simulink model "b10_wp_snake"  (R2021b)
settings: Solver=VariableStepAuto  StartTime=0.0  StopTime=Inf  FixedStep=sampleTime  RelTol=1e-3  EnableMultiTasking=on
InitFcn:
  | sampleTime = 0.05;
  | nMedianSize=3;
  | % Robot parameters
  | % Robot parameters
  | wheelRadius = 0.0303;
  | robotRadius = 0.07;   %小车在仿真中显示的圆形的半径大小
  | Trackwidth = 0.0847;  %定义向量场直方图算法中小车的宽度
  | 
  | % Lidar parameters
  | sensorOffset = [0,0];
  | scanAngles = linspace(-pi/3,pi/3,20)';%y = linspace(x1,x2,n) 生成 n 个点。这些点的间距为 (x2-x1)/(n-1)。
  | maxRange = 0.2;
  | 
  | %%%%%%
  | ks=1;
  | 
  | init_pose_1=[0    0  0]';
  | init_pose_2=[0    0.2  -pi/2]';
  | init_pose_3=[0    0.4  -pi/2]';
  | init_pose_4=[0    0.6  -pi/2]';
  | init_pose_5=[0    0.8  -pi/2]';
  | init_pose_6=[0    1  -pi/2]';
  | init_pose_7=[0    1.2  -pi/2]';
  | init_pose_8=[0    1.4  -pi/2]';
  | init_pose_9=[0    1.6  -pi/2]';
  | init_pose_10=[0   1.8  -pi/2]';
  | 
  | % paremeters of pure persuit
  | desired_v=0.2;
  | desired_w=2*pi;
  | desired_lookahead=0.2;
  | kv=0;
  | kw=1;%加速转弯
  | GoalRadius=0.15;%到达目标判定阈值
  | 
  | % paremeters of recovery
  | %recovery_w=0.5
  | recovery_w=2;
  | % Vector Field Histogram
  | numSector=180;%Number of angular sector
  | vehicleRadius=robotRadius;
  | rangeDis=[ 0, 0 ];%Range distance limits (m):
  | thresholds=[ 3, 8 ];%Histogram thresholds
  | %binary histogram 大于8是障碍物，小于3是空白区
  | %Thresholds for computing binary histogram, specified as a two-element vector of scalars. The algorithm uses these thresholds to compute the binary histogram from the polar obstacle density. Polar obstacle density values higher than the upper threshold are represented as occupied space (1) in the binary histogram. Values smaller than the lower threshold are represented as free space (0). Values that fall between the limits are set to the values of a previous computed binary histogram if one exists from previous iterations. If a previous histogram does not exist, the value is set as free space (0).
  | safetyDis=0.1;%Safety distance
  | minimumTurningRadius=0.5*robotRadius;%Minimum turning radius (m):
undefined symbols (not defined in the file): Angular, DiscIntNeverNeededParam, Linear, Pose, Twist
libraries: robotlib x72, dspstat3 x30, mobileRoboticsLib x21, robotalgslib x20, robotmobilelib x10
(part 1 of 6)
settings Model: Creator=The MathWorks, Inc.  LastModifiedBy=FCS
settings SolverCC: AlgebraicLoopSolver=TrustRegion
settings DataIOCC: LimitDataPoints=on  SaveFormat=Array  ReturnWorkspaceOutputs=off
settings OptimizationCC: EnhancedBackFolding=on  PassReuseOutputArgsAs=Individual arguments  ZeroExternalMemoryAtStartup=off  ZeroInternalMemoryAtStartup=off  MaxStackSize=64  OptimizeBlockOrder=speed  DifferentSizesBufferReuse=on  OptimizationCustomize=off  EfficientTunableParamExpr=on
settings DebuggingCC: SolverPrmCheckMsg=warning  ParameterTunabilityLossMsg=error  SFUnexpectedBacktrackingDiag=warning  SFNoUnconditionalDefaultTransitionDiag=warning  SFExecutionAtInitializationDiag=none  SFMachineParentedDataDiag=warning  ArithmeticOperatorsInVariantConditions=warning
settings HardwareCC: ProdBitPerPointer=32  ProdBitPerSizeT=32  ProdBitPerPtrDiffT=32  ProdLargestAtomicFloat=None  ProdIntDivRoundTo=Undefined  ProdEndianess=Unspecified  ProdWordSize=32  ProdHWDeviceType=Generic->Unspecified (assume 32-bit Generic)  TargetHWDeviceType=Generic->Unspecified (assume 32-bit Generic)
settings ModelReferenceCC: PropagateSignalLabelsOutOfModel=off
settings SFSimCC: SimUseLocalCustomCode=off  CustomCodeUndefinedFunction=UseInterfaceOnly  SimTargetLang=C++
settings RTWCC: Description=Embedded Coder  SystemTargetFile=ert.tlc  HardwareBoard=Robot Operating System (ROS)  TLCOptions="-aInlineSetEventsForThisBaseRateFcn=TLC_FALSE -aSuppressMultiTaskScheduler=TLC_FALSE  -aRateBasedStepFcn=0"  TemplateMakefile=ert_default_tmf  RTWUseLocalCustomCode=off  Toolchain=Catkin  TargetLang=C++
settings CodeAppCC: ForceParamTrailComments=on  IgnoreCustomStorageClasses=off  OperatorAnnotations=on  SimulinkDataObjDesc=on  SFDataObjDesc=on  InsertBlockDesc=on
settings ERTTargetCC: SupportVariableSizeSignals=on
settings ConfigComp: CovMetricSettings=dw  CovSaveCumulativeToWorkspaceVar=on  CovSaveSingleToWorkspaceVar=on  CovExternalEMLEnable=off  CovSFcnEnable=off

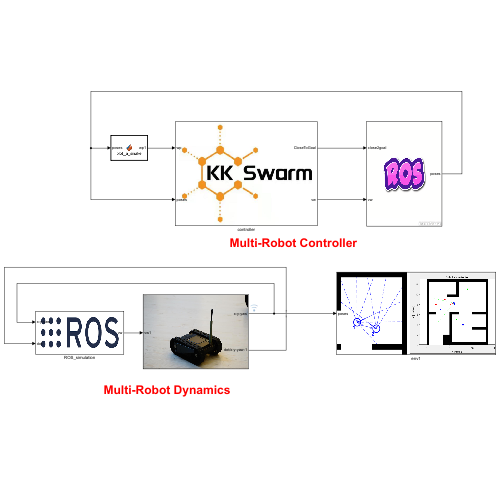
[thumbnail: Simulink's stored preview of the top-level diagram]
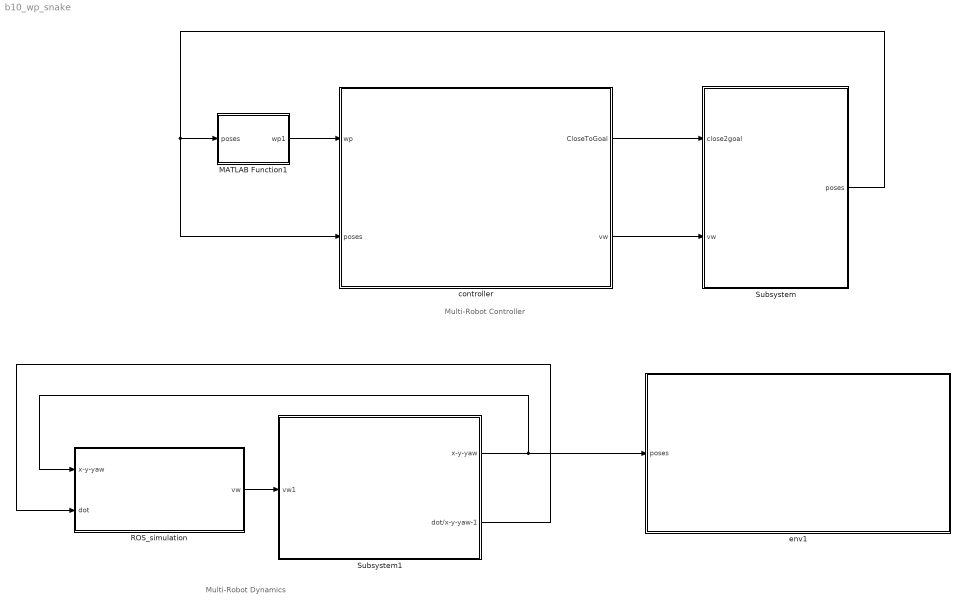
== system b10_wp_snake ==
  note: Multi-Robot Controller
  note: Multi-Robot Dynamics
  MATLAB Function1 : MATLAB Function  TreatAsAtomicUnit=on
  ROS_simulation : Subsystem
      mask Display: image('$imagefile'); % 使用工具条上的 "编辑图像" 进行更改。
  Subsystem : Subsystem
      mask Display: image('$imagefile'); % 使用工具条上的 "编辑图像" 进行更改。
  Subsystem1 : Subsystem
      mask Display: image('$imagefile'); % 使用工具条上的 "编辑图像" 进行更改。
  controller : Subsystem
      mask Display: image('$imagefile'); % 使用工具条上的 "编辑图像" 进行更改。
  env1 : Subsystem
      mask Display: image('$imagefile'); % 使用工具条上的 "编辑图像" 进行更改。
  wires:
  controller/1(CloseToGoal) -> Subsystem/1(close2goal)
  controller/2(vw) -> Subsystem/2(vw)
  Subsystem/1(poses) -> MATLAB Function1/1(poses), controller/2(poses)
  MATLAB Function1/1(wp1) -> controller/1(wp)
  ROS_simulation/1(vw) -> Subsystem1/1(vw1)
  Subsystem1/2(dot/x-y-yaw-1) -> ROS_simulation/2(dot)
  Subsystem1/1(x-y-yaw) -> env1/1(poses), ROS_simulation/1(x-y-yaw)

== system b10_wp_snake/ROS_simulation ==
  x-y-yaw : Inport
  dot : Inport  Port=2
  Demux1 : Demux  Outputs=10
  Demux3 : Demux  Outputs=10
  Mux6 : Mux  Inputs=10
  ros1 : Subsystem
  ros10 : Subsystem
  ros2 : Subsystem
  ros3 : Subsystem
  ros4 : Subsystem
  ros5 : Subsystem
  ros6 : Subsystem
  ros7 : Subsystem
  ros8 : Subsystem
  ros9 : Subsystem
  vw : Outport
  wires:
  ros5/1(vw1) -> Mux6/5
  ros2/1(vw1) -> Mux6/2
  ros3/1(vw1) -> Mux6/3
  ros4/1(vw1) -> Mux6/4
  ros1/1(vw1) -> Mux6/1
  ros6/1(vw1) -> Mux6/6
  ros7/1(vw1) -> Mux6/7
  ros8/1(vw1) -> Mux6/8
  ros9/1(vw1) -> Mux6/9
  Mux6/1 -> vw/1
  ros10/1(vw1) -> Mux6/10
  Demux1/1 -> ros1/1(x-y-yaw1)
  Demux1/2 -> ros2/1(x-y-yaw1)
  Demux1/3 -> ros3/1(x-y-yaw1)
  Demux1/4 -> ros4/1(x-y-yaw1)
  Demux1/5 -> ros5/1(x-y-yaw1)
  Demux1/6 -> ros6/1(x-y-yaw1)
  Demux1/7 -> ros7/1(x-y-yaw1)
  Demux1/8 -> ros8/1(x-y-yaw1)
  Demux1/9 -> ros9/1(x-y-yaw1)
  Demux1/10 -> ros10/1(x-y-yaw1)
  Demux3/1 -> ros1/2(do1t)
  Demux3/2 -> ros2/2(dot)
  Demux3/3 -> ros3/2(do1t)
  Demux3/4 -> ros4/2(do1t)
  Demux3/5 -> ros5/2(do1t)
  Demux3/6 -> ros6/2(do1t)
  Demux3/7 -> ros7/2(do1t)
  Demux3/8 -> ros8/2(do1t)
  Demux3/9 -> ros9/2(do1t)
  Demux3/10 -> ros10/2(do1t)
  x-y-yaw/1 -> Demux1/1
  dot/1 -> Demux3/1

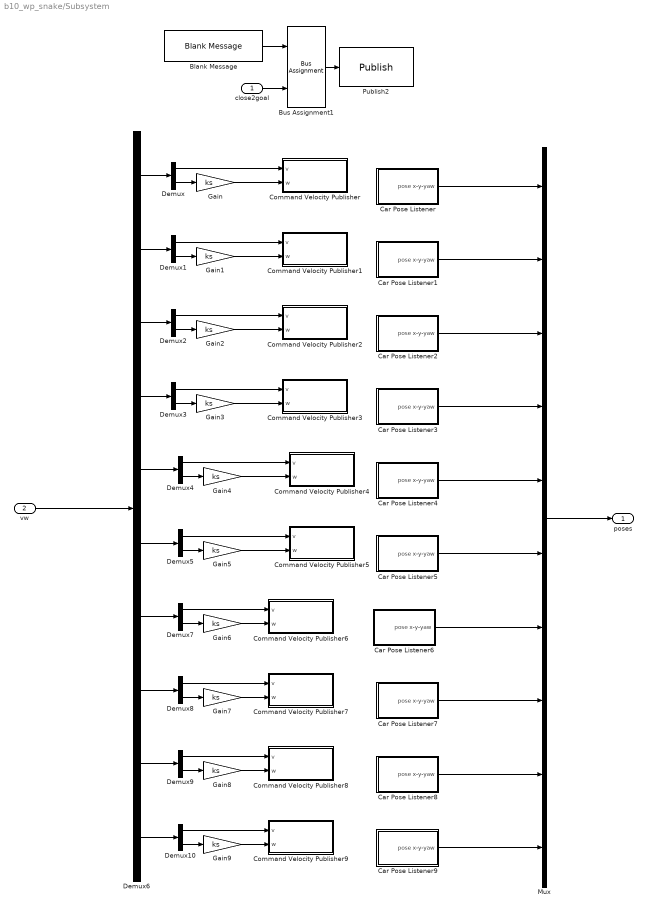
== system b10_wp_snake/Subsystem ==
  close2goal : Inport
  vw : Inport  Port=2
  Blank Message : robotlib/Blank Message  messageClass=Message  entityType=std_msgs/Float64  messageType=std_msgs/Float64  SampleTime=inf  legacyBusStruct=off
  Bus Assignment1 : BusAssignment  DialogController=Simulink.DDGSource_BusAssignment  AssignedSignals=Data
  Car Pose Listener : Subsystem
  Car Pose Listener1 : Subsystem
  Car Pose Listener2 : Subsystem
  Car Pose Listener3 : Subsystem
  Car Pose Listener4 : Subsystem
  Car Pose Listener5 : Subsystem
  Car Pose Listener6 : Subsystem
  Car Pose Listener7 : Subsystem
  Car Pose Listener8 : Subsystem
  Car Pose Listener9 : Subsystem
  Command Velocity Publisher : Subsystem
  Command Velocity Publisher1 : Subsystem
  Command Velocity Publisher2 : Subsystem
  Command Velocity Publisher3 : Subsystem
  Command Velocity Publisher4 : Subsystem
  Command Velocity Publisher5 : Subsystem
  Command Velocity Publisher6 : Subsystem
  Command Velocity Publisher7 : Subsystem
  Command Velocity Publisher8 : Subsystem
  Command Velocity Publisher9 : Subsystem
  Demux{,1..5,7..10} (10 alike) : Demux  Outputs=2
  Demux6 : Demux  Outputs=10
  Gain{,1..9} (10 alike) : Gain  Gain=ks
  Mux : Mux  Inputs=10
  Publish2 : robotlib/Publish  topicSource=Specify your own  topic=/close_goal  messageType=std_msgs/Float64  legacyBusStruct=off  messageQueueLength=105
  poses : Outport
  wires:
  Gain/1 -> Command Velocity Publisher/2(w)
  Demux/2 -> Gain/1
  Car Pose Listener/1(pose x-y-yaw) -> Mux/1
  Demux/1 -> Command Velocity Publisher/1(v)
  Car Pose Listener1/1(pose x-y-yaw) -> Mux/2
  Gain1/1 -> Command Velocity Publisher1/2(w)
  Demux1/2 -> Gain1/1
  Demux1/1 -> Command Velocity Publisher1/1(v)
  Car Pose Listener2/1(pose x-y-yaw) -> Mux/3
  Gain2/1 -> Command Velocity Publisher2/2(w)
  Demux2/2 -> Gain2/1
  Demux2/1 -> Command Velocity Publisher2/1(v)
  Car Pose Listener3/1(pose x-y-yaw) -> Mux/4
  Gain3/1 -> Command Velocity Publisher3/2(w)
  Demux3/2 -> Gain3/1
  Demux3/1 -> Command Velocity Publisher3/1(v)
  Gain4/1 -> Command Velocity Publisher4/2(w)
  Demux6/5 -> Demux4/1
  Demux4/2 -> Gain4/1
  Demux4/1 -> Command Velocity Publisher4/1(v)
  Car Pose Listener5/1(pose x-y-yaw) -> Mux/6
  Gain5/1 -> Command Velocity Publisher5/2(w)
  Demux6/6 -> Demux5/1
  Demux5/2 -> Gain5/1
  Demux5/1 -> Command Velocity Publisher5/1(v)
  Bus Assignment1/1 -> Publish2/1
  Blank Message/1 -> Bus Assignment1/1
  close2goal/1 -> Bus Assignment1/2
  Demux6/1 -> Demux/1
  Demux6/2 -> Demux1/1
  Demux6/3 -> Demux2/1
  Demux6/4 -> Demux3/1
  Car Pose Listener6/1(pose x-y-yaw) -> Mux/7
  Demux7/1 -> Command Velocity Publisher6/1(v)
  Demux7/2 -> Gain6/1
  Gain6/1 -> Command Velocity Publisher6/2(w)
  Demux6/7 -> Demux7/1
  Car Pose Listener7/1(pose x-y-yaw) -> Mux/8
  Demux8/1 -> Command Velocity Publisher7/1(v)
  Demux8/2 -> Gain7/1
  Gain7/1 -> Command Velocity Publisher7/2(w)
  Demux6/8 -> Demux8/1
  Car Pose Listener8/1(pose x-y-yaw) -> Mux/9
  Demux9/1 -> Command Velocity Publisher8/1(v)
  Demux9/2 -> Gain8/1
  Gain8/1 -> Command Velocity Publisher8/2(w)
  Demux6/9 -> Demux9/1
  Car Pose Listener9/1(pose x-y-yaw) -> Mux/10
  Demux10/1 -> Command Velocity Publisher9/1(v)
  Demux10/2 -> Gain9/1
  Gain9/1 -> Command Velocity Publisher9/2(w)
  Demux6/10 -> Demux10/1
  vw/1 -> Demux6/1
  Car Pose Listener4/1(pose x-y-yaw) -> Mux/5
  Mux/1 -> poses/1

== system b10_wp_snake/Subsystem1 ==
  vw1 : Inport
  Demux1 : Demux  Outputs=10
  Mux1 : Mux  Inputs=10
  Mux6 : Mux  Inputs=10
  car_model1 : Subsystem
  car_model10 : Subsystem
  car_model2 : Subsystem
  car_model3 : Subsystem
  car_model4 : Subsystem
  car_model5 : Subsystem
  car_model6 : Subsystem
  car_model7 : Subsystem
  car_model8 : Subsystem
  car_model9 : Subsystem
  x-y-yaw : Outport
  dot/x-y-yaw-1 : Outport  Port=2
  wires:
  Demux1/1 -> car_model1/1(vw1)
  Demux1/2 -> car_model2/1(vw1)
  vw1/1 -> Demux1/1
  Demux1/3 -> car_model3/1(vw1)
  Demux1/4 -> car_model4/1(vw1)
  Demux1/5 -> car_model5/1(vw1)
  Demux1/6 -> car_model6/1(vw1)
  Demux1/7 -> car_model7/1(vw1)
  Demux1/8 -> car_model8/1(vw1)
  Demux1/9 -> car_model9/1(vw1)
  Mux6/1 -> dot/x-y-yaw-1/1
  Demux1/10 -> car_model10/1(vw1)
  Mux1/1 -> x-y-yaw/1
  car_model10/1(x-y-yaw) -> Mux1/10
  car_model9/1(x-y-yaw) -> Mux1/9
  car_model8/1(x-y-yaw) -> Mux1/8
  car_model7/1(x-y-yaw) -> Mux1/7
  car_model6/1(x-y-yaw) -> Mux1/6
  car_model5/1(x-y-yaw) -> Mux1/5
  car_model1/1(x-y-yaw) -> Mux1/1
  car_model2/1(x-y-yaw) -> Mux1/2
  car_model3/1(x-y-yaw) -> Mux1/3
  car_model4/1(x-y-yaw) -> Mux1/4
  car_model1/2(dot) -> Mux6/1
  car_model2/2(dot) -> Mux6/2
  car_model3/2(dot) -> Mux6/3
  car_model4/2(dot) -> Mux6/4
  car_model5/2(dot) -> Mux6/5
  car_model6/2(dot) -> Mux6/6
  car_model7/2(dot) -> Mux6/7
  car_model8/2(dot) -> Mux6/8
  car_model9/2(dot) -> Mux6/9
  car_model10/2(dot) -> Mux6/10

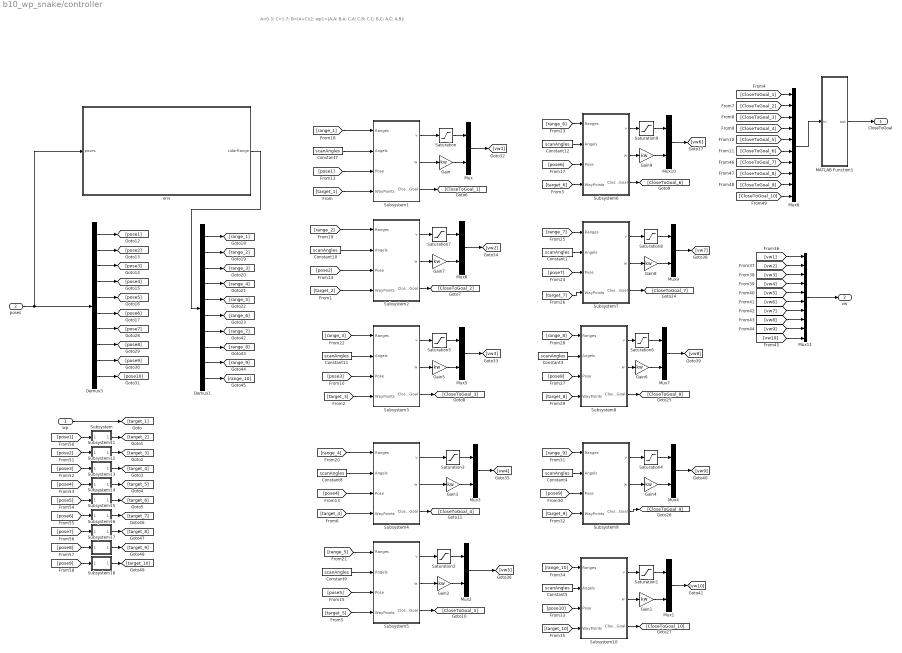
== system b10_wp_snake/controller ==
  note: A=0.3;
      | C=1.7;
      | B=(A+C)/2;
      |
      | wp1=[A,A; B,A; C,A;
      | C,B;
      | C,C; B,C; A,C;
      | A,B];
  wp : Inport
  poses : Inport  Port=2
  Constant{1,3..5,7..12} (10 alike) : Constant  Value=scanAngles
  Demux1 : Demux  Outputs=10
  Demux3 : Demux  Outputs=10
  Gain{,1..9} (10 alike) : Gain  Gain=kw
  MATLAB Function1 : MATLAB Function  TreatAsAtomicUnit=on
  Mux{,1..5,7..10} (10 alike) : Mux  Inputs=2
  Mux11 : Mux  Inputs=10
  Mux6 : Mux  Inputs=10
  Saturation{,1..9} (10 alike) : Saturate  UpperLimit=1  LowerLimit=0
  Subsystem : Subsystem
  Subsystem1 : Subsystem
  Subsystem10 : Subsystem
  Subsystem11 : Subsystem
  Subsystem12 : Subsystem
  Subsystem13 : Subsystem
  Subsystem14 : Subsystem
  Subsystem15 : Subsystem
  Subsystem16 : Subsystem
  Subsystem17 : Subsystem
  Subsystem18 : Subsystem
  Subsystem2 : Subsystem
  Subsystem3 : Subsystem
  Subsystem4 : Subsystem
  Subsystem5 : Subsystem
  Subsystem6 : Subsystem
  Subsystem7 : Subsystem
  Subsystem8 : Subsystem
  Subsystem9 : Subsystem
  env : Subsystem
      mask Display: image('$imagefile'); % 使用工具条上的 "编辑图像" 进行更改。
  CloseToGoal : Outport
  vw : Outport  Port=2
  wires:
  [pose3] -> Subsystem12/1(In1)
  [range_3] -> Subsystem3/1(Ranges)
  Subsystem4/3(CloseToGoal) -> [CloseToGoal_4]
  [pose1] -> Subsystem/1(In1)
  Saturation/1 -> Mux/1
  Subsystem1/3(CloseToGoal) -> [CloseToGoal_1]
  Subsystem3/3(CloseToGoal) -> [CloseToGoal_3]
  Subsystem5/3(CloseToGoal) -> [CloseToGoal_5]
  Subsystem6/3(CloseToGoal) -> [CloseToGoal_6]
  [target_3] -> Subsystem3/4(WayPoints)
  Subsystem2/3(CloseToGoal) -> [CloseToGoal_2]
  Constant10/1 -> Subsystem2/2(Angels)
  [pose2] -> Subsystem2/3(Pose)
  Constant7/1 -> Subsystem1/2(Angels)
  Constant11/1 -> Subsystem3/2(Angels)
  [range_6] -> Subsystem6/1(Ranges)
  wp/1 -> [target_1]
  [pose2] -> Subsystem11/1(In1)
  [pose4] -> Subsystem13/1(In1)
  Constant9/1 -> Subsystem5/2(Angels)
  [target_6] -> Subsystem6/4(WayPoints)
  [pose5] -> Subsystem14/1(In1)
  Gain/1 -> Mux/2
  [pose5] -> Subsystem5/3(Pose)
  [pose3] -> Subsystem3/3(Pose)
  [target_4] -> Subsystem4/4(WayPoints)
  [range_4] -> Subsystem4/1(Ranges)
  Constant8/1 -> Subsystem4/2(Angels)
  Constant12/1 -> Subsystem6/2(Angels)
  [target_2] -> Subsystem2/4(WayPoints)
  [target_1] -> Subsystem1/4(WayPoints)
  Subsystem1/1(v) -> Saturation/1
  [target_5] -> Subsystem5/4(WayPoints)
  [range_5] -> Subsystem5/1(Ranges)
  [pose6] -> Subsystem6/3(Pose)
  [pose1] -> Subsystem1/3(Pose)
  Mux/1 -> [vw1]
  [pose4] -> Subsystem4/3(Pose)
  [CloseToGoal_2] -> Mux6/2
  [CloseToGoal_6] -> Mux6/6
  [CloseToGoal_3] -> Mux6/3
  [CloseToGoal_1] -> Mux6/1
  MATLAB Function1/1(out) -> CloseToGoal/1
  Mux6/1 -> MATLAB Function1/1(in)
  [CloseToGoal_4] -> Mux6/4
  [CloseToGoal_5] -> Mux6/5
  Demux3/3 -> [pose3]
  Demux3/6 -> [pose6]
  Demux3/1 -> [pose1]
  Demux3/5 -> [pose5]
  Demux3/2 -> [pose2]
  Demux3/4 -> [pose4]
  poses/1 -> Demux3/1, env/1(poses)
  Demux1/3 -> [range_3]
  Demux1/2 -> [range_2]
  Demux1/1 -> [range_1]
  Demux1/4 -> [range_4]
  Demux1/6 -> [range_6]
  Demux1/5 -> [range_5]
  env/1(LidarRange) -> Demux1/1
  [range_1] -> Subsystem1/1(Ranges)
  [range_2] -> Subsystem2/1(Ranges)
  [range_7] -> Subsystem7/1(Ranges)
  Constant1/1 -> Subsystem7/2(Angels)
  [target_7] -> Subsystem7/4(WayPoints)
  Subsystem7/3(CloseToGoal) -> [CloseToGoal_7]
  [pose7] -> Subsystem7/3(Pose)
  [range_8] -> Subsystem8/1(Ranges)
  Constant3/1 -> Subsystem8/2(Angels)
  [target_8] -> Subsystem8/4(WayPoints)
  Subsystem8/3(CloseToGoal) -> [CloseToGoal_8]
  [pose8] -> Subsystem8/3(Pose)
  [range_9] -> Subsystem9/1(Ranges)
  Constant4/1 -> Subsystem9/2(Angels)
  [target_9] -> Subsystem9/4(WayPoints)
  Subsystem9/3(CloseToGoal) -> [CloseToGoal_9]
  [range_10] -> Subsystem10/1(Ranges)
  Constant5/1 -> Subsystem10/2(Angels)
  [target_10] -> Subsystem10/4(WayPoints)
  Subsystem10/3(CloseToGoal) -> [CloseToGoal_10]
  [pose10] -> Subsystem10/3(Pose)
  Demux3/7 -> [pose7]
  Demux3/8 -> [pose8]
  Demux3/9 -> [pose9]
  Demux3/10 -> [pose10]
  [vw1] -> Mux11/1
  [vw2] -> Mux11/2
  [vw3] -> Mux11/3
  [vw4] -> Mux11/4
  [vw5] -> Mux11/5
  [vw6] -> Mux11/6
  [vw7] -> Mux11/7
  [vw8] -> Mux11/8
  [vw9] -> Mux11/9
  [vw10] -> Mux11/10
  Mux11/1 -> vw/1
  Demux1/7 -> [range_7]
  Demux1/8 -> [range_8]
  Demux1/9 -> [range_9]
  Demux1/10 -> [range_10]
  [pose6] -> Subsystem15/1(In1)
  [pose7] -> Subsystem16/1(In1)
  [pose8] -> Subsystem17/1(In1)
  [pose9] -> Subsystem18/1(In1)
  [pose9] -> Subsystem9/3(Pose)
  Subsystem1/2(w) -> Gain/1
  [CloseToGoal_7] -> Mux6/7
  [CloseToGoal_9] -> Mux6/9
  [CloseToGoal_10] -> Mux6/10
  [CloseToGoal_8] -> Mux6/8
  Gain1/1 -> Mux1/2
  Mux1/1 -> [vw10]
  Saturation1/1 -> Mux1/1
  Subsystem10/1(v) -> Saturation1/1
  Subsystem10/2(w) -> Gain1/1
  Gain2/1 -> Mux2/2
  Mux2/1 -> [vw5]
  Saturation2/1 -> Mux2/1
  Subsystem5/1(v) -> Saturation2/1
  Subsystem5/2(w) -> Gain2/1
  Gain3/1 -> Mux3/2
  Mux3/1 -> [vw4]
  Saturation3/1 -> Mux3/1
  Subsystem4/1(v) -> Saturation3/1
  Subsystem4/2(w) -> Gain3/1
  Gain4/1 -> Mux4/2
  Mux4/1 -> [vw9]
  Saturation4/1 -> Mux4/1
  Subsystem9/1(v) -> Saturation4/1
  Subsystem9/2(w) -> Gain4/1
  Gain5/1 -> Mux5/2
  Mux5/1 -> [vw3]
  Saturation5/1 -> Mux5/1
  Subsystem3/1(v) -> Saturation5/1
  Subsystem3/2(w) -> Gain5/1
  Gain6/1 -> Mux7/2
  Mux7/1 -> [vw8]
  Saturation6/1 -> Mux7/1
  Subsystem8/1(v) -> Saturation6/1
  Subsystem8/2(w) -> Gain6/1
  Gain7/1 -> Mux8/2
  Mux8/1 -> [vw2]
  Saturation7/1 -> Mux8/1
  Subsystem2/1(v) -> Saturation7/1
  Subsystem2/2(w) -> Gain7/1
  Gain8/1 -> Mux9/2
  Mux9/1 -> [vw7]
  Saturation8/1 -> Mux9/1
  Subsystem7/1(v) -> Saturation8/1
  Subsystem7/2(w) -> Gain8/1
  Gain9/1 -> Mux10/2
  Mux10/1 -> [vw6]
  Saturation9/1 -> Mux10/1
  Subsystem6/1(v) -> Saturation9/1
  Subsystem6/2(w) -> Gain9/1
  Subsystem/1(Out1) -> [target_2]
  Subsystem11/1(Out1) -> [target_3]
  Subsystem12/1(Out1) -> [target_4]
  Subsystem13/1(Out1) -> [target_5]
  Subsystem14/1(Out1) -> [target_6]
  Subsystem15/1(Out1) -> [target_7]
  Subsystem16/1(Out1) -> [target_8]
  Subsystem17/1(Out1) -> [target_9]
  Subsystem18/1(Out1) -> [target_10]

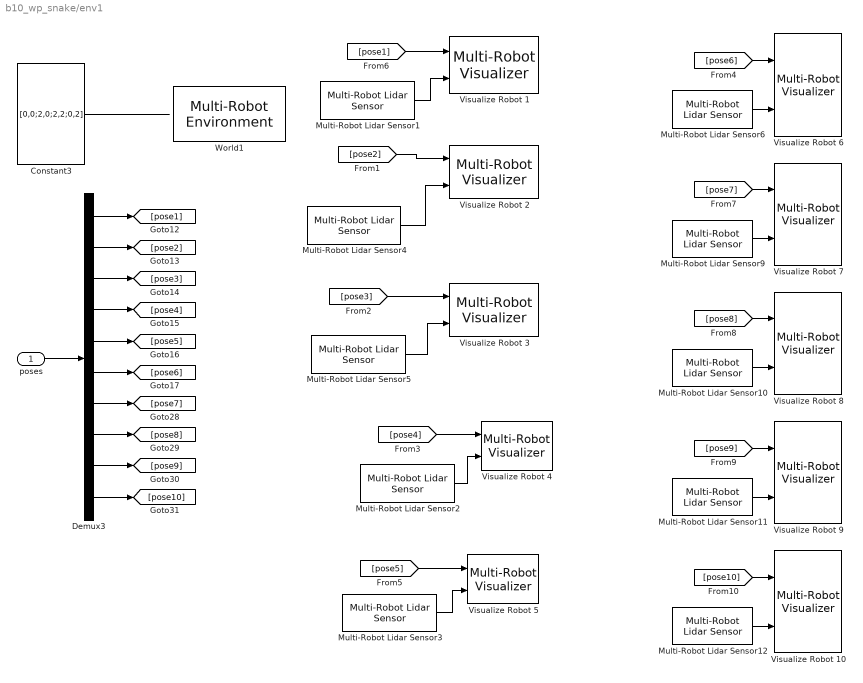
== system b10_wp_snake/env1 ==
  poses : Inport
  Constant3 : Constant  Value=[0,0;2,0;2,2;0,2]
  Demux3 : Demux  Outputs=10
  Multi-Robot Lidar Sensor1 : mobileRoboticsLib/Environments/Multi-Robot Lidar Sensor  robotIdx=1  sensorOffset=sensorOffset  scanAngles=scanAngles  maxRange=maxRange
      settings: SourceProductName=Mobile Robotics Simulation Toolbox
  Multi-Robot Lidar Sensor10 : mobileRoboticsLib/Environments/Multi-Robot Lidar Sensor  robotIdx=8  sensorOffset=sensorOffset  scanAngles=scanAngles  maxRange=maxRange
      settings: SourceProductName=Mobile Robotics Simulation Toolbox
  Multi-Robot Lidar Sensor11 : mobileRoboticsLib/Environments/Multi-Robot Lidar Sensor  robotIdx=9  sensorOffset=sensorOffset  scanAngles=scanAngles  maxRange=maxRange
      settings: SourceProductName=Mobile Robotics Simulation Toolbox
  Multi-Robot Lidar Sensor12 : mobileRoboticsLib/Environments/Multi-Robot Lidar Sensor  robotIdx=10  sensorOffset=sensorOffset  scanAngles=scanAngles  maxRange=maxRange
      settings: SourceProductName=Mobile Robotics Simulation Toolbox
  Multi-Robot Lidar Sensor2 : mobileRoboticsLib/Environments/Multi-Robot Lidar Sensor  robotIdx=4  sensorOffset=sensorOffset  scanAngles=scanAngles  maxRange=maxRange
      settings: SourceProductName=Mobile Robotics Simulation Toolbox
  Multi-Robot Lidar Sensor3 : mobileRoboticsLib/Environments/Multi-Robot Lidar Sensor  robotIdx=5  sensorOffset=sensorOffset  scanAngles=scanAngles  maxRange=maxRange
      settings: SourceProductName=Mobile Robotics Simulation Toolbox
  Multi-Robot Lidar Sensor4 : mobileRoboticsLib/Environments/Multi-Robot Lidar Sensor  robotIdx=2  sensorOffset=sensorOffset  scanAngles=scanAngles  maxRange=maxRange
      settings: SourceProductName=Mobile Robotics Simulation Toolbox
  Multi-Robot Lidar Sensor5 : mobileRoboticsLib/Environments/Multi-Robot Lidar Sensor  robotIdx=3  sensorOffset=sensorOffset  scanAngles=scanAngles  maxRange=maxRange
      settings: SourceProductName=Mobile Robotics Simulation Toolbox
  Multi-Robot Lidar Sensor6 : mobileRoboticsLib/Environments/Multi-Robot Lidar Sensor  robotIdx=6  sensorOffset=sensorOffset  scanAngles=scanAngles  maxRange=maxRange
      settings: SourceProductName=Mobile Robotics Simulation Toolbox
  Multi-Robot Lidar Sensor9 : mobileRoboticsLib/Environments/Multi-Robot Lidar Sensor  robotIdx=7  sensorOffset=sensorOffset  scanAngles=scanAngles  maxRange=maxRange
      settings: SourceProductName=Mobile Robotics Simulation Toolbox
  Visualize Robot 1 : mobileRoboticsLib/Environments/Multi-Robot Visualizer  idx=1  radius=robotRadius  robotColor=[0 0 1]  showTraj=off  hasLidar=on  sensorOffset=sensorOffset  scanAngles=scanAngles  maxNumScans=0  hasObjDetector=off  objDetectorOffset=[0,0]  objDetectorAngle=0  objDetectorFOV=pi/2  objDetectorMaxRange=5  hasRobotDetector=off  robotDetectorOffset=[0,0]  robotDetectorAngle=0  robotDetectorFOV=pi/3  robotDetectorMaxRange=5  robotDetectorNumDetections=0
      settings: SourceProductName=Mobile Robotics Simulation Toolbox
  Visualize Robot 10 : mobileRoboticsLib/Environments/Multi-Robot Visualizer  idx=10  radius=robotRadius  robotColor=[1 0 0]  showTraj=off  hasLidar=on  sensorOffset=sensorOffset  scanAngles=scanAngles  maxNumScans=0  hasObjDetector=off  objDetectorOffset=[0,0]  objDetectorAngle=0  objDetectorFOV=pi/2  objDetectorMaxRange=5  hasRobotDetector=off  robotDetectorOffset=[0,0]  robotDetectorAngle=0  robotDetectorFOV=pi/3  robotDetectorMaxRange=5  robotDetectorNumDetections=0
      settings: SourceProductName=Mobile Robotics Simulation Toolbox
  Visualize Robot 2 : mobileRoboticsLib/Environments/Multi-Robot Visualizer  idx=2  radius=robotRadius  robotColor=[0 1 0]  showTraj=on  hasLidar=on  sensorOffset=sensorOffset  scanAngles=scanAngles  maxNumScans=0  hasObjDetector=off  objDetectorOffset=[0,0]  objDetectorAngle=0  objDetectorFOV=pi/2  objDetectorMaxRange=5  hasRobotDetector=off  robotDetectorOffset=[0,0]  robotDetectorAngle=0  robotDetectorFOV=pi/3  robotDetectorMaxRange=5  robotDetectorNumDetections=0
      settings: SourceProductName=Mobile Robotics Simulation Toolbox
  Visualize Robot 3 : mobileRoboticsLib/Environments/Multi-Robot Visualizer  idx=3  radius=robotRadius  robotColor=[0 1 0]  showTraj=off  hasLidar=on  sensorOffset=sensorOffset  scanAngles=scanAngles  maxNumScans=0  hasObjDetector=off  objDetectorOffset=[0,0]  objDetectorAngle=0  objDetectorFOV=pi/2  objDetectorMaxRange=5  hasRobotDetector=off  robotDetectorOffset=[0,0]  robotDetectorAngle=0  robotDetectorFOV=pi/3  robotDetectorMaxRange=5  robotDetectorNumDetections=0
      settings: SourceProductName=Mobile Robotics Simulation Toolbox
  Visualize Robot 4 : mobileRoboticsLib/Environments/Multi-Robot Visualizer  idx=4  radius=robotRadius  robotColor=[1 0 0]  showTraj=on  hasLidar=on  sensorOffset=sensorOffset  scanAngles=scanAngles  maxNumScans=0  hasObjDetector=off  objDetectorOffset=[0,0]  objDetectorAngle=0  objDetectorFOV=pi/2  objDetectorMaxRange=5  hasRobotDetector=off  robotDetectorOffset=[0,0]  robotDetectorAngle=0  robotDetectorFOV=pi/3  robotDetectorMaxRange=5  robotDetectorNumDetections=0
      settings: SourceProductName=Mobile Robotics Simulation Toolbox
  Visualize Robot 5 : mobileRoboticsLib/Environments/Multi-Robot Visualizer  idx=5  radius=robotRadius  robotColor=[1 0 1]  showTraj=off  hasLidar=on  sensorOffset=sensorOffset  scanAngles=scanAngles  maxNumScans=0  hasObjDetector=off  objDetectorOffset=[0,0]  objDetectorAngle=0  objDetectorFOV=pi/2  objDetectorMaxRange=5  hasRobotDetector=off  robotDetectorOffset=[0,0]  robotDetectorAngle=0  robotDetectorFOV=pi/3  robotDetectorMaxRange=5  robotDetectorNumDetections=0
      settings: SourceProductName=Mobile Robotics Simulation Toolbox
  Visualize Robot 6 : mobileRoboticsLib/Environments/Multi-Robot Visualizer  idx=6  radius=robotRadius  robotColor=[1 0 0]  showTraj=off  hasLidar=on  sensorOffset=sensorOffset  scanAngles=scanAngles  maxNumScans=0  hasObjDetector=off  objDetectorOffset=[0,0]  objDetectorAngle=0  objDetectorFOV=pi/2  objDetectorMaxRange=5  hasRobotDetector=off  robotDetectorOffset=[0,0]  robotDetectorAngle=0  robotDetectorFOV=pi/3  robotDetectorMaxRange=5  robotDetectorNumDetections=0
      settings: SourceProductName=Mobile Robotics Simulation Toolbox
  Visualize Robot 7 : mobileRoboticsLib/Environments/Multi-Robot Visualizer  idx=7  radius=robotRadius  robotColor=[1 0 0]  showTraj=off  hasLidar=on  sensorOffset=sensorOffset  scanAngles=scanAngles  maxNumScans=0  hasObjDetector=off  objDetectorOffset=[0,0]  objDetectorAngle=0  objDetectorFOV=pi/2  objDetectorMaxRange=5  hasRobotDetector=off  robotDetectorOffset=[0,0]  robotDetectorAngle=0  robotDetectorFOV=pi/3  robotDetectorMaxRange=5  robotDetectorNumDetections=0
      settings: SourceProductName=Mobile Robotics Simulation Toolbox
  Visualize Robot 8 : mobileRoboticsLib/Environments/Multi-Robot Visualizer  idx=8  radius=robotRadius  robotColor=[1 0 0]  showTraj=off  hasLidar=on  sensorOffset=sensorOffset  scanAngles=scanAngles  maxNumScans=0  hasObjDetector=off  objDetectorOffset=[0,0]  objDetectorAngle=0  objDetectorFOV=pi/2  objDetectorMaxRange=5  hasRobotDetector=off  robotDetectorOffset=[0,0]  robotDetectorAngle=0  robotDetectorFOV=pi/3  robotDetectorMaxRange=5  robotDetectorNumDetections=0
      settings: SourceProductName=Mobile Robotics Simulation Toolbox
  Visualize Robot 9 : mobileRoboticsLib/Environments/Multi-Robot Visualizer  idx=9  radius=robotRadius  robotColor=[1 0 0]  showTraj=off  hasLidar=on  sensorOffset=sensorOffset  scanAngles=scanAngles  maxNumScans=0  hasObjDetector=off  objDetectorOffset=[0,0]  objDetectorAngle=0  objDetectorFOV=pi/2  objDetectorMaxRange=5  hasRobotDetector=off  robotDetectorOffset=[0,0]  robotDetectorAngle=0  robotDetectorFOV=pi/3  robotDetectorMaxRange=5  robotDetectorNumDetections=0
      settings: SourceProductName=Mobile Robotics Simulation Toolbox
  World1 : mobileRoboticsLib/Environments/Multi-Robot Environment  numRobots=10  showWaypoints=on  showObjects=off  objectColors=[1 0 0;0 1 0;0 0 1]  objectMarkers='s'  showRobotIds=on  plotSensorLines=on
      settings: SourceProductName=Mobile Robotics Simulation Toolbox
  wires:
  poses/1 -> Demux3/1
  Multi-Robot Lidar Sensor12/1 -> Visualize Robot 10/2
  [pose10] -> Visualize Robot 10/1
  Multi-Robot Lidar Sensor11/1 -> Visualize Robot 9/2
  [pose9] -> Visualize Robot 9/1
  Multi-Robot Lidar Sensor10/1 -> Visualize Robot 8/2
  [pose8] -> Visualize Robot 8/1
  Multi-Robot Lidar Sensor9/1 -> Visualize Robot 7/2
  [pose7] -> Visualize Robot 7/1
  Demux3/1 -> [pose1]
  Demux3/7 -> [pose7]
  Demux3/9 -> [pose9]
  Demux3/8 -> [pose8]
  Demux3/6 -> [pose6]
  Demux3/4 -> [pose4]
  Demux3/2 -> [pose2]
  Demux3/3 -> [pose3]
  Demux3/5 -> [pose5]
  Demux3/10 -> [pose10]
  [pose3] -> Visualize Robot 3/1
  Multi-Robot Lidar Sensor3/1 -> Visualize Robot 5/2
  [pose5] -> Visualize Robot 5/1
  [pose4] -> Visualize Robot 4/1
  [pose1] -> Visualize Robot 1/1
  [pose6] -> Visualize Robot 6/1
  Multi-Robot Lidar Sensor2/1 -> Visualize Robot 4/2
  Multi-Robot Lidar Sensor6/1 -> Visualize Robot 6/2
  Multi-Robot Lidar Sensor1/1 -> Visualize Robot 1/2
  [pose2] -> Visualize Robot 2/1
  Multi-Robot Lidar Sensor4/1 -> Visualize Robot 2/2
  Multi-Robot Lidar Sensor5/1 -> Visualize Robot 3/2
  Constant3/1 -> ?

== system b10_wp_snake/ROS_simulation/ros1 ==
  x-y-yaw1 : Inport
  do1t : Inport  Port=2
  " [x y theta]" : Demux  Outputs=3
  " [x y theta]1" : Demux  Outputs=3
  Blank Message : robotlib/Blank Message  messageClass=Message  entityType=nav_msgs/Odometry  messageType=nav_msgs/Odometry  SampleTime=inf  legacyBusStruct=off
  Bus Assignment1 : BusAssignment  DialogController=Simulink.DDGSource_BusAssignment  AssignedSignals=Pose.Pose.Position.X,Pose.Pose.Position.Y,Pose.Pose.Orientation.Z,Pose.Pose.Orientation.W,Twist.Twist.Linear.X,Twist.Twist.Linear.Y,Twist.Twist.Angular.Z
  Bus Selector3 : BusSelector  OutputSignals=Linear.X,Angular.Z
  MATLAB Function : MATLAB Function  TreatAsAtomicUnit=on
  Mux5 : Mux  Inputs=2
  Publish2 : robotlib/Publish  topicSource=Specify your own  topic=/robot_1/pose  messageType=nav_msgs/Odometry  legacyBusStruct=off  messageQueueLength=105
  Subscribe1 : robotlib/Subscribe  topicSource=Specify your own  topic=/robot_1/cmd_vel  messageType=geometry_msgs/Twist  SampleTime=-1  legacyBusStruct=off  messageQueueLength=51
  Terminator : Terminator
  Terminator1 : Terminator
  Zero-Order Hold : ZeroOrderHold  SampleTime=0.1
  Zero-Order Hold1 : ZeroOrderHold  SampleTime=0.1
  vw1 : Outport
  wires:
  " [x y theta]"/1 -> Bus Assignment1/2
  Blank Message/1 -> Bus Assignment1/1
  x-y-yaw1/1 -> Zero-Order Hold/1
  " [x y theta]"/2 -> Bus Assignment1/3
  " [x y theta]1"/2 -> Bus Assignment1/7
  " [x y theta]"/3 -> MATLAB Function/1(yaw)
  " [x y theta]1"/3 -> Bus Assignment1/8
  MATLAB Function/4(w) -> Bus Assignment1/5
  MATLAB Function/3(z) -> Bus Assignment1/4
  " [x y theta]1"/1 -> Bus Assignment1/6
  Bus Assignment1/1 -> Publish2/1
  do1t/1 -> Zero-Order Hold1/1
  MATLAB Function/1(x) -> Terminator/1
  MATLAB Function/2(y) -> Terminator1/1
  Bus Selector3/1 -> Mux5/1  "<X>"
  Bus Selector3/2 -> Mux5/2  "<Z>"
  Subscribe1/2 -> Bus Selector3/1
  Mux5/1 -> vw1/1
  Zero-Order Hold/1 -> " [x y theta]"/1
  Zero-Order Hold1/1 -> " [x y theta]1"/1

== system b10_wp_snake/ROS_simulation/ros10 ==
  x-y-yaw1 : Inport
  do1t : Inport  Port=2
  " [x y theta]" : Demux  Outputs=3
  " [x y theta]1" : Demux  Outputs=3
  Blank Message : robotlib/Blank Message  messageClass=Message  entityType=nav_msgs/Odometry  messageType=nav_msgs/Odometry  SampleTime=inf  legacyBusStruct=off
  Bus Assignment1 : BusAssignment  DialogController=Simulink.DDGSource_BusAssignment  AssignedSignals=Pose.Pose.Position.X,Pose.Pose.Position.Y,Pose.Pose.Orientation.Z,Pose.Pose.Orientation.W,Twist.Twist.Linear.X,Twist.Twist.Linear.Y,Twist.Twist.Angular.Z
  Bus Selector3 : BusSelector  OutputSignals=Linear.X,Angular.Z
  MATLAB Function : MATLAB Function  TreatAsAtomicUnit=on
  Mux5 : Mux  Inputs=2
  Publish2 : robotlib/Publish  topicSource=Specify your own  topic=/robot_10/pose  messageType=nav_msgs/Odometry  legacyBusStruct=off  messageQueueLength=105
  Subscribe1 : robotlib/Subscribe  topicSource=Specify your own  topic=/robot_10/cmd_vel  messageType=geometry_msgs/Twist  SampleTime=-1  legacyBusStruct=off  messageQueueLength=51
  Terminator : Terminator
  Terminator1 : Terminator
  Zero-Order Hold : ZeroOrderHold  SampleTime=0.1
  Zero-Order Hold1 : ZeroOrderHold  SampleTime=0.1
  vw1 : Outport
  wires:
  " [x y theta]"/1 -> Bus Assignment1/2
  Blank Message/1 -> Bus Assignment1/1
  x-y-yaw1/1 -> Zero-Order Hold/1
  " [x y theta]"/2 -> Bus Assignment1/3
  " [x y theta]1"/2 -> Bus Assignment1/7
  " [x y theta]"/3 -> MATLAB Function/1(yaw)
  " [x y theta]1"/3 -> Bus Assignment1/8
  MATLAB Function/4(w) -> Bus Assignment1/5
  MATLAB Function/3(z) -> Bus Assignment1/4
  " [x y theta]1"/1 -> Bus Assignment1/6
  Bus Assignment1/1 -> Publish2/1
  do1t/1 -> Zero-Order Hold1/1
  MATLAB Function/1(x) -> Terminator/1
  MATLAB Function/2(y) -> Terminator1/1
  Bus Selector3/1 -> Mux5/1  "<X>"
  Bus Selector3/2 -> Mux5/2  "<Z>"
  Subscribe1/2 -> Bus Selector3/1
  Mux5/1 -> vw1/1
  Zero-Order Hold/1 -> " [x y theta]"/1
  Zero-Order Hold1/1 -> " [x y theta]1"/1

== system b10_wp_snake/ROS_simulation/ros2 ==
  x-y-yaw1 : Inport
  dot : Inport  Port=2
  " [x y theta]" : Demux  Outputs=3
  " [x y theta]1" : Demux  Outputs=3
  Blank Message : robotlib/Blank Message  messageClass=Message  entityType=nav_msgs/Odometry  messageType=nav_msgs/Odometry  SampleTime=inf  legacyBusStruct=off
  Bus Assignment1 : BusAssignment  DialogController=Simulink.DDGSource_BusAssignment  AssignedSignals=Pose.Pose.Position.X,Pose.Pose.Position.Y,Pose.Pose.Orientation.Z,Pose.Pose.Orientation.W,Twist.Twist.Linear.X,Twist.Twist.Linear.Y,Twist.Twist.Angular.Z
  Bus Selector3 : BusSelector  OutputSignals=Linear.X,Angular.Z
  MATLAB Function : MATLAB Function  TreatAsAtomicUnit=on
  Mux5 : Mux  Inputs=2
  Publish2 : robotlib/Publish  topicSource=Specify your own  topic=/robot_2/pose  messageType=nav_msgs/Odometry  legacyBusStruct=off  messageQueueLength=105
  Subscribe1 : robotlib/Subscribe  topicSource=Specify your own  topic=/robot_2/cmd_vel  messageType=geometry_msgs/Twist  SampleTime=-1  legacyBusStruct=off  messageQueueLength=51
  Terminator : Terminator
  Terminator1 : Terminator
  Zero-Order Hold : ZeroOrderHold  SampleTime=0.1
  Zero-Order Hold1 : ZeroOrderHold  SampleTime=0.1
  vw1 : Outport
  wires:
  " [x y theta]"/1 -> Bus Assignment1/2
  Blank Message/1 -> Bus Assignment1/1
  x-y-yaw1/1 -> Zero-Order Hold/1
  " [x y theta]"/2 -> Bus Assignment1/3
  " [x y theta]1"/2 -> Bus Assignment1/7
  " [x y theta]"/3 -> MATLAB Function/1(yaw)
  " [x y theta]1"/3 -> Bus Assignment1/8
  MATLAB Function/4(w) -> Bus Assignment1/5
  MATLAB Function/3(z) -> Bus Assignment1/4
  " [x y theta]1"/1 -> Bus Assignment1/6
  Bus Assignment1/1 -> Publish2/1
  dot/1 -> Zero-Order Hold1/1
  MATLAB Function/1(x) -> Terminator/1
  MATLAB Function/2(y) -> Terminator1/1
  Bus Selector3/1 -> Mux5/1  "<X>"
  Bus Selector3/2 -> Mux5/2  "<Z>"
  Subscribe1/2 -> Bus Selector3/1
  Mux5/1 -> vw1/1
  Zero-Order Hold/1 -> " [x y theta]"/1
  Zero-Order Hold1/1 -> " [x y theta]1"/1

== system b10_wp_snake/ROS_simulation/ros3 ==
  x-y-yaw1 : Inport
  do1t : Inport  Port=2
  " [x y theta]" : Demux  Outputs=3
  " [x y theta]1" : Demux  Outputs=3
  Blank Message : robotlib/Blank Message  messageClass=Message  entityType=nav_msgs/Odometry  messageType=nav_msgs/Odometry  SampleTime=inf  legacyBusStruct=off
  Bus Assignment1 : BusAssignment  DialogController=Simulink.DDGSource_BusAssignment  AssignedSignals=Pose.Pose.Position.X,Pose.Pose.Position.Y,Pose.Pose.Orientation.Z,Pose.Pose.Orientation.W,Twist.Twist.Linear.X,Twist.Twist.Linear.Y,Twist.Twist.Angular.Z
  Bus Selector3 : BusSelector  OutputSignals=Linear.X,Angular.Z
  MATLAB Function : MATLAB Function  TreatAsAtomicUnit=on
  Mux5 : Mux  Inputs=2
  Publish2 : robotlib/Publish  topicSource=Specify your own  topic=/robot_3/pose  messageType=nav_msgs/Odometry  legacyBusStruct=off  messageQueueLength=105
  Subscribe1 : robotlib/Subscribe  topicSource=Specify your own  topic=/robot_3/cmd_vel  messageType=geometry_msgs/Twist  SampleTime=-1  legacyBusStruct=off  messageQueueLength=51
  Terminator : Terminator
  Terminator1 : Terminator
  Zero-Order Hold : ZeroOrderHold  SampleTime=0.1
  Zero-Order Hold1 : ZeroOrderHold  SampleTime=0.1
  vw1 : Outport
  wires:
  " [x y theta]"/1 -> Bus Assignment1/2
  Blank Message/1 -> Bus Assignment1/1
  x-y-yaw1/1 -> Zero-Order Hold/1
  " [x y theta]"/2 -> Bus Assignment1/3
  " [x y theta]1"/2 -> Bus Assignment1/7
  " [x y theta]"/3 -> MATLAB Function/1(yaw)
  " [x y theta]1"/3 -> Bus Assignment1/8
  MATLAB Function/4(w) -> Bus Assignment1/5
  MATLAB Function/3(z) -> Bus Assignment1/4
  " [x y theta]1"/1 -> Bus Assignment1/6
  Bus Assignment1/1 -> Publish2/1
  do1t/1 -> Zero-Order Hold1/1
  MATLAB Function/1(x) -> Terminator/1
  MATLAB Function/2(y) -> Terminator1/1
  Bus Selector3/1 -> Mux5/1  "<X>"
  Bus Selector3/2 -> Mux5/2  "<Z>"
  Subscribe1/2 -> Bus Selector3/1
  Mux5/1 -> vw1/1
  Zero-Order Hold/1 -> " [x y theta]"/1
  Zero-Order Hold1/1 -> " [x y theta]1"/1

== system b10_wp_snake/ROS_simulation/ros4 ==
  x-y-yaw1 : Inport
  do1t : Inport  Port=2
  " [x y theta]" : Demux  Outputs=3
  " [x y theta]1" : Demux  Outputs=3
  Blank Message : robotlib/Blank Message  messageClass=Message  entityType=nav_msgs/Odometry  messageType=nav_msgs/Odometry  SampleTime=inf  legacyBusStruct=off
  Bus Assignment1 : BusAssignment  DialogController=Simulink.DDGSource_BusAssignment  AssignedSignals=Pose.Pose.Position.X,Pose.Pose.Position.Y,Pose.Pose.Orientation.Z,Pose.Pose.Orientation.W,Twist.Twist.Linear.X,Twist.Twist.Linear.Y,Twist.Twist.Angular.Z
  Bus Selector3 : BusSelector  OutputSignals=Linear.X,Angular.Z
  MATLAB Function : MATLAB Function  TreatAsAtomicUnit=on
  Mux5 : Mux  Inputs=2
  Publish2 : robotlib/Publish  topicSource=Specify your own  topic=/robot_4/pose  messageType=nav_msgs/Odometry  legacyBusStruct=off  messageQueueLength=105
  Subscribe1 : robotlib/Subscribe  topicSource=Specify your own  topic=/robot_4/cmd_vel  messageType=geometry_msgs/Twist  SampleTime=-1  legacyBusStruct=off  messageQueueLength=51
  Terminator : Terminator
  Terminator1 : Terminator
  Zero-Order Hold : ZeroOrderHold  SampleTime=0.1
  Zero-Order Hold1 : ZeroOrderHold  SampleTime=0.1
  vw1 : Outport
  wires:
  " [x y theta]"/1 -> Bus Assignment1/2
  Blank Message/1 -> Bus Assignment1/1
  x-y-yaw1/1 -> Zero-Order Hold/1
  " [x y theta]"/2 -> Bus Assignment1/3
  " [x y theta]1"/2 -> Bus Assignment1/7
  " [x y theta]"/3 -> MATLAB Function/1(yaw)
  " [x y theta]1"/3 -> Bus Assignment1/8
  MATLAB Function/4(w) -> Bus Assignment1/5
  MATLAB Function/3(z) -> Bus Assignment1/4
  " [x y theta]1"/1 -> Bus Assignment1/6
  Bus Assignment1/1 -> Publish2/1
  do1t/1 -> Zero-Order Hold1/1
  MATLAB Function/1(x) -> Terminator/1
  MATLAB Function/2(y) -> Terminator1/1
  Bus Selector3/1 -> Mux5/1  "<X>"
  Bus Selector3/2 -> Mux5/2  "<Z>"
  Subscribe1/2 -> Bus Selector3/1
  Mux5/1 -> vw1/1
  Zero-Order Hold/1 -> " [x y theta]"/1
  Zero-Order Hold1/1 -> " [x y theta]1"/1

== system b10_wp_snake/ROS_simulation/ros5 ==
  x-y-yaw1 : Inport
  do1t : Inport  Port=2
  " [x y theta]" : Demux  Outputs=3
  " [x y theta]1" : Demux  Outputs=3
  Blank Message : robotlib/Blank Message  messageClass=Message  entityType=nav_msgs/Odometry  messageType=nav_msgs/Odometry  SampleTime=inf  legacyBusStruct=off
  Bus Assignment1 : BusAssignment  DialogController=Simulink.DDGSource_BusAssignment  AssignedSignals=Pose.Pose.Position.X,Pose.Pose.Position.Y,Pose.Pose.Orientation.Z,Pose.Pose.Orientation.W,Twist.Twist.Linear.X,Twist.Twist.Linear.Y,Twist.Twist.Angular.Z
  Bus Selector3 : BusSelector  OutputSignals=Linear.X,Angular.Z
  MATLAB Function : MATLAB Function  TreatAsAtomicUnit=on
  Mux5 : Mux  Inputs=2
  Publish2 : robotlib/Publish  topicSource=Specify your own  topic=/robot_5/pose  messageType=nav_msgs/Odometry  legacyBusStruct=off  messageQueueLength=105
  Subscribe1 : robotlib/Subscribe  topicSource=Specify your own  topic=/robot_5/cmd_vel  messageType=geometry_msgs/Twist  SampleTime=-1  legacyBusStruct=off  messageQueueLength=51
  Terminator : Terminator
  Terminator1 : Terminator
  Zero-Order Hold : ZeroOrderHold  SampleTime=0.1
  Zero-Order Hold1 : ZeroOrderHold  SampleTime=0.1
  vw1 : Outport
  wires:
  " [x y theta]"/1 -> Bus Assignment1/2
  Blank Message/1 -> Bus Assignment1/1
  x-y-yaw1/1 -> Zero-Order Hold/1
  " [x y theta]"/2 -> Bus Assignment1/3
  " [x y theta]1"/2 -> Bus Assignment1/7
  " [x y theta]"/3 -> MATLAB Function/1(yaw)
  " [x y theta]1"/3 -> Bus Assignment1/8
  MATLAB Function/4(w) -> Bus Assignment1/5
  MATLAB Function/3(z) -> Bus Assignment1/4
  " [x y theta]1"/1 -> Bus Assignment1/6
  Bus Assignment1/1 -> Publish2/1
  do1t/1 -> Zero-Order Hold1/1
  MATLAB Function/1(x) -> Terminator/1
  MATLAB Function/2(y) -> Terminator1/1
  Bus Selector3/1 -> Mux5/1  "<X>"
  Bus Selector3/2 -> Mux5/2  "<Z>"
  Subscribe1/2 -> Bus Selector3/1
  Mux5/1 -> vw1/1
  Zero-Order Hold/1 -> " [x y theta]"/1
  Zero-Order Hold1/1 -> " [x y theta]1"/1

== system b10_wp_snake/ROS_simulation/ros6 ==
  x-y-yaw1 : Inport
  do1t : Inport  Port=2
  " [x y theta]" : Demux  Outputs=3
  " [x y theta]1" : Demux  Outputs=3
  Blank Message : robotlib/Blank Message  messageClass=Message  entityType=nav_msgs/Odometry  messageType=nav_msgs/Odometry  SampleTime=inf  legacyBusStruct=off
  Bus Assignment1 : BusAssignment  DialogController=Simulink.DDGSource_BusAssignment  AssignedSignals=Pose.Pose.Position.X,Pose.Pose.Position.Y,Pose.Pose.Orientation.Z,Pose.Pose.Orientation.W,Twist.Twist.Linear.X,Twist.Twist.Linear.Y,Twist.Twist.Angular.Z
  Bus Selector3 : BusSelector  OutputSignals=Linear.X,Angular.Z
  MATLAB Function : MATLAB Function  TreatAsAtomicUnit=on
  Mux5 : Mux  Inputs=2
  Publish2 : robotlib/Publish  topicSource=Specify your own  topic=/robot_6/pose  messageType=nav_msgs/Odometry  legacyBusStruct=off  messageQueueLength=105
  Subscribe1 : robotlib/Subscribe  topicSource=Specify your own  topic=/robot_6/cmd_vel  messageType=geometry_msgs/Twist  SampleTime=-1  legacyBusStruct=off  messageQueueLength=51
  Terminator : Terminator
  Terminator1 : Terminator
  Zero-Order Hold : ZeroOrderHold  SampleTime=0.1
  Zero-Order Hold1 : ZeroOrderHold  SampleTime=0.1
  vw1 : Outport
  wires:
  " [x y theta]"/1 -> Bus Assignment1/2
  Blank Message/1 -> Bus Assignment1/1
  x-y-yaw1/1 -> Zero-Order Hold/1
  " [x y theta]"/2 -> Bus Assignment1/3
  " [x y theta]1"/2 -> Bus Assignment1/7
  " [x y theta]"/3 -> MATLAB Function/1(yaw)
  " [x y theta]1"/3 -> Bus Assignment1/8
  MATLAB Function/4(w) -> Bus Assignment1/5
  MATLAB Function/3(z) -> Bus Assignment1/4
  " [x y theta]1"/1 -> Bus Assignment1/6
  Bus Assignment1/1 -> Publish2/1
  do1t/1 -> Zero-Order Hold1/1
  MATLAB Function/1(x) -> Terminator/1
  MATLAB Function/2(y) -> Terminator1/1
  Bus Selector3/1 -> Mux5/1  "<X>"
  Bus Selector3/2 -> Mux5/2  "<Z>"
  Subscribe1/2 -> Bus Selector3/1
  Mux5/1 -> vw1/1
  Zero-Order Hold/1 -> " [x y theta]"/1
  Zero-Order Hold1/1 -> " [x y theta]1"/1

== system b10_wp_snake/ROS_simulation/ros7 ==
  x-y-yaw1 : Inport
  do1t : Inport  Port=2
  " [x y theta]" : Demux  Outputs=3
  " [x y theta]1" : Demux  Outputs=3
  Blank Message : robotlib/Blank Message  messageClass=Message  entityType=nav_msgs/Odometry  messageType=nav_msgs/Odometry  SampleTime=inf  legacyBusStruct=off
  Bus Assignment1 : BusAssignment  DialogController=Simulink.DDGSource_BusAssignment  AssignedSignals=Pose.Pose.Position.X,Pose.Pose.Position.Y,Pose.Pose.Orientation.Z,Pose.Pose.Orientation.W,Twist.Twist.Linear.X,Twist.Twist.Linear.Y,Twist.Twist.Angular.Z
  Bus Selector3 : BusSelector  OutputSignals=Linear.X,Angular.Z
  MATLAB Function : MATLAB Function  TreatAsAtomicUnit=on
  Mux5 : Mux  Inputs=2
  Publish2 : robotlib/Publish  topicSource=Specify your own  topic=/robot_7/pose  messageType=nav_msgs/Odometry  legacyBusStruct=off  messageQueueLength=105
  Subscribe1 : robotlib/Subscribe  topicSource=Specify your own  topic=/robot_7/cmd_vel  messageType=geometry_msgs/Twist  SampleTime=-1  legacyBusStruct=off  messageQueueLength=51
  Terminator : Terminator
  Terminator1 : Terminator
  Zero-Order Hold : ZeroOrderHold  SampleTime=0.1
  Zero-Order Hold1 : ZeroOrderHold  SampleTime=0.1
  vw1 : Outport
  wires:
  " [x y theta]"/1 -> Bus Assignment1/2
  Blank Message/1 -> Bus Assignment1/1
  x-y-yaw1/1 -> Zero-Order Hold/1
  " [x y theta]"/2 -> Bus Assignment1/3
  " [x y theta]1"/2 -> Bus Assignment1/7
  " [x y theta]"/3 -> MATLAB Function/1(yaw)
  " [x y theta]1"/3 -> Bus Assignment1/8
  MATLAB Function/4(w) -> Bus Assignment1/5
  MATLAB Function/3(z) -> Bus Assignment1/4
  " [x y theta]1"/1 -> Bus Assignment1/6
  Bus Assignment1/1 -> Publish2/1
  do1t/1 -> Zero-Order Hold1/1
  MATLAB Function/1(x) -> Terminator/1
  MATLAB Function/2(y) -> Terminator1/1
  Bus Selector3/1 -> Mux5/1  "<X>"
  Bus Selector3/2 -> Mux5/2  "<Z>"
  Subscribe1/2 -> Bus Selector3/1
  Mux5/1 -> vw1/1
  Zero-Order Hold/1 -> " [x y theta]"/1
  Zero-Order Hold1/1 -> " [x y theta]1"/1

== system b10_wp_snake/ROS_simulation/ros8 ==
  x-y-yaw1 : Inport
  do1t : Inport  Port=2
  " [x y theta]" : Demux  Outputs=3
  " [x y theta]1" : Demux  Outputs=3
  Blank Message : robotlib/Blank Message  messageClass=Message  entityType=nav_msgs/Odometry  messageType=nav_msgs/Odometry  SampleTime=inf  legacyBusStruct=off
  Bus Assignment1 : BusAssignment  DialogController=Simulink.DDGSource_BusAssignment  AssignedSignals=Pose.Pose.Position.X,Pose.Pose.Position.Y,Pose.Pose.Orientation.Z,Pose.Pose.Orientation.W,Twist.Twist.Linear.X,Twist.Twist.Linear.Y,Twist.Twist.Angular.Z
  Bus Selector3 : BusSelector  OutputSignals=Linear.X,Angular.Z
  MATLAB Function : MATLAB Function  TreatAsAtomicUnit=on
  Mux5 : Mux  Inputs=2
  Publish2 : robotlib/Publish  topicSource=Specify your own  topic=/robot_8/pose  messageType=nav_msgs/Odometry  legacyBusStruct=off  messageQueueLength=105
  Subscribe1 : robotlib/Subscribe  topicSource=Specify your own  topic=/robot_8/cmd_vel  messageType=geometry_msgs/Twist  SampleTime=-1  legacyBusStruct=off  messageQueueLength=51
  Terminator : Terminator
  Terminator1 : Terminator
  Zero-Order Hold : ZeroOrderHold  SampleTime=0.1
  Zero-Order Hold1 : ZeroOrderHold  SampleTime=0.1
  vw1 : Outport
  wires:
  " [x y theta]"/1 -> Bus Assignment1/2
  Blank Message/1 -> Bus Assignment1/1
  x-y-yaw1/1 -> Zero-Order Hold/1
  " [x y theta]"/2 -> Bus Assignment1/3
  " [x y theta]1"/2 -> Bus Assignment1/7
  " [x y theta]"/3 -> MATLAB Function/1(yaw)
  " [x y theta]1"/3 -> Bus Assignment1/8
  MATLAB Function/4(w) -> Bus Assignment1/5
  MATLAB Function/3(z) -> Bus Assignment1/4
  " [x y theta]1"/1 -> Bus Assignment1/6
  Bus Assignment1/1 -> Publish2/1
  do1t/1 -> Zero-Order Hold1/1
  MATLAB Function/1(x) -> Terminator/1
  MATLAB Function/2(y) -> Terminator1/1
  Bus Selector3/1 -> Mux5/1  "<X>"
  Bus Selector3/2 -> Mux5/2  "<Z>"
  Subscribe1/2 -> Bus Selector3/1
  Mux5/1 -> vw1/1
  Zero-Order Hold/1 -> " [x y theta]"/1
  Zero-Order Hold1/1 -> " [x y theta]1"/1

== system b10_wp_snake/ROS_simulation/ros9 ==
  x-y-yaw1 : Inport
  do1t : Inport  Port=2
  " [x y theta]" : Demux  Outputs=3
  " [x y theta]1" : Demux  Outputs=3
  Blank Message : robotlib/Blank Message  messageClass=Message  entityType=nav_msgs/Odometry  messageType=nav_msgs/Odometry  SampleTime=inf  legacyBusStruct=off
  Bus Assignment1 : BusAssignment  DialogController=Simulink.DDGSource_BusAssignment  AssignedSignals=Pose.Pose.Position.X,Pose.Pose.Position.Y,Pose.Pose.Orientation.Z,Pose.Pose.Orientation.W,Twist.Twist.Linear.X,Twist.Twist.Linear.Y,Twist.Twist.Angular.Z
  Bus Selector3 : BusSelector  OutputSignals=Linear.X,Angular.Z
  MATLAB Function : MATLAB Function  TreatAsAtomicUnit=on
  Mux5 : Mux  Inputs=2
  Publish2 : robotlib/Publish  topicSource=Specify your own  topic=/robot_9/pose  messageType=nav_msgs/Odometry  legacyBusStruct=off  messageQueueLength=105
  Subscribe1 : robotlib/Subscribe  topicSource=Specify your own  topic=/robot_9/cmd_vel  messageType=geometry_msgs/Twist  SampleTime=-1  legacyBusStruct=off  messageQueueLength=51
  Terminator : Terminator
  Terminator1 : Terminator
  Zero-Order Hold : ZeroOrderHold  SampleTime=0.1
  Zero-Order Hold1 : ZeroOrderHold  SampleTime=0.1
  vw1 : Outport
  wires:
  " [x y theta]"/1 -> Bus Assignment1/2
  Blank Message/1 -> Bus Assignment1/1
  x-y-yaw1/1 -> Zero-Order Hold/1
  " [x y theta]"/2 -> Bus Assignment1/3
  " [x y theta]1"/2 -> Bus Assignment1/7
  " [x y theta]"/3 -> MATLAB Function/1(yaw)
  " [x y theta]1"/3 -> Bus Assignment1/8
  MATLAB Function/4(w) -> Bus Assignment1/5
  MATLAB Function/3(z) -> Bus Assignment1/4
  " [x y theta]1"/1 -> Bus Assignment1/6
  Bus Assignment1/1 -> Publish2/1
  do1t/1 -> Zero-Order Hold1/1
  MATLAB Function/1(x) -> Terminator/1
  MATLAB Function/2(y) -> Terminator1/1
  Bus Selector3/1 -> Mux5/1  "<X>"
  Bus Selector3/2 -> Mux5/2  "<Z>"
  Subscribe1/2 -> Bus Selector3/1
  Mux5/1 -> vw1/1
  Zero-Order Hold/1 -> " [x y theta]"/1
  Zero-Order Hold1/1 -> " [x y theta]1"/1

== system b10_wp_snake/Subsystem/Car Pose Listener ==
  Subscribe : robotlib/Subscribe  topicSource=Specify your own  topic=/robot_1/pose  messageType=nav_msgs/Odometry  SampleTime=-1  legacyBusStruct=off  messageQueueLength=51
  Subscribe1 : robotlib/Subscribe  topicSource=Specify your own  topic=/robot_1/odometry  messageType=geometry_msgs/Twist  SampleTime=-1  legacyBusStruct=off  messageQueueLength=51
  Subsystem : Subsystem
  pose x-y-yaw : Outport
  wires:
  Subscribe/1 -> Subsystem/1(poseNew)  "IsNew"
  Subscribe/2 -> Subsystem/2(poseMsg)
  Subscribe1/1 -> Subsystem/3(VW_New)  "IsNew"
  Subscribe1/2 -> Subsystem/4(VW_Msg)
  Subsystem/1(pose) -> pose x-y-yaw/1

== system b10_wp_snake/Subsystem/Car Pose Listener1 ==
  Subscribe : robotlib/Subscribe  topicSource=Specify your own  topic=/robot_2/pose  messageType=nav_msgs/Odometry  SampleTime=-1  legacyBusStruct=off  messageQueueLength=51
  Subscribe1 : robotlib/Subscribe  topicSource=Specify your own  topic=/robot_2/odometry  messageType=geometry_msgs/Twist  SampleTime=-1  legacyBusStruct=off  messageQueueLength=51
  Subsystem : Subsystem
  pose x-y-yaw : Outport
  wires:
  Subscribe/1 -> Subsystem/1(poseNew)  "IsNew"
  Subscribe/2 -> Subsystem/2(poseMsg)
  Subscribe1/2 -> Subsystem/4(VW_Msg)
  Subscribe1/1 -> Subsystem/3(VW_New)  "IsNew"
  Subsystem/1(pose) -> pose x-y-yaw/1

== system b10_wp_snake/Subsystem/Car Pose Listener2 ==
  Subscribe : robotlib/Subscribe  topicSource=Specify your own  topic=/robot_3/pose  messageType=nav_msgs/Odometry  SampleTime=-1  legacyBusStruct=off  messageQueueLength=51
  Subscribe1 : robotlib/Subscribe  topicSource=Specify your own  topic=/robot_3/odometry  messageType=geometry_msgs/Twist  SampleTime=-1  legacyBusStruct=off  messageQueueLength=51
  Subsystem : Subsystem
  pose x-y-yaw : Outport
  wires:
  Subscribe/1 -> Subsystem/1(poseNew)  "IsNew"
  Subscribe/2 -> Subsystem/2(poseMsg)
  Subscribe1/1 -> Subsystem/3(VW_New)  "IsNew"
  Subscribe1/2 -> Subsystem/4(VW_Msg)
  Subsystem/1(pose) -> pose x-y-yaw/1

== system b10_wp_snake/Subsystem/Car Pose Listener3 ==
  Subscribe : robotlib/Subscribe  topicSource=Specify your own  topic=/robot_4/pose  messageType=nav_msgs/Odometry  SampleTime=-1  legacyBusStruct=off  messageQueueLength=51
  Subscribe1 : robotlib/Subscribe  topicSource=Specify your own  topic=/robot_4/odometry  messageType=geometry_msgs/Twist  SampleTime=-1  legacyBusStruct=off  messageQueueLength=51
  Subsystem : Subsystem
  pose x-y-yaw : Outport
  wires:
  Subscribe/1 -> Subsystem/1(poseNew)  "IsNew"
  Subscribe/2 -> Subsystem/2(poseMsg)
  Subscribe1/1 -> Subsystem/3(VW_New)  "IsNew"
  Subscribe1/2 -> Subsystem/4(VW_Msg)
  Subsystem/1(pose) -> pose x-y-yaw/1
